simulink model "UpDownPendulum"  (Simulink 8.6)
settings: Solver=ode1  SolverMode=SingleTasking  StartTime=0.0  StopTime=200  FixedStep=0.001  RelTol=1e-3
undefined symbols (not defined in the file): Advantech, magnitude, PCI
libraries: sldrtlib x11, simulink x6
settings Model: Creator=Demo11  LastModifiedBy=demo  SimulationMode=external  ExtModeTrigMode=oneshot  ExtModeTrigDuration=100000
settings DataIOCC: LimitDataPoints=off  SignalLoggingName=sigsOut
settings OptimizationCC: BlockReduction=off  BooleanDataType=off  InitFltsAndDblsToZero=on
settings DebuggingCC: SaveWithParameterizedLinksMsg=none  SignalResolutionControl=TryResolveAllWithWarning  SolverPrmCheckMsg=none  MultiTaskDSMMsg=warning  MultiTaskCondExecSysMsg=none  FcnCallInpInsideContextMsg=UseLocalSettings
settings HardwareCC: ProdBitPerLong=64  ProdBitPerPointer=64  ProdIntDivRoundTo=Zero  ProdEndianess=LittleEndian  ProdWordSize=64  ProdHWDeviceType=Intel->x86-64  TargetBitPerLong=64  TargetBitPerPointer=64  TargetIntDivRoundTo=Zero  TargetEndianess=LittleEndian  TargetWordSize=64  TargetHWDeviceType=Intel->x86-64
settings RTWCC: SystemTargetFile=sldrt.tlc  TemplateMakefile=sldrt.tmf  Description=Simulink Desktop Real-Time  RTWCompilerOptimization=on
settings CodeAppCC: MaxIdLength=95
settings SimulinkDesktopRealTimeCC: TargetPreCompLibLocation=C:\Program Files\MATLAB\R2015b\toolbox\sldrt\lib\win64  TargetLangStandard=C89/C90 (ANSI)  SupportVariableSizeSignals=off

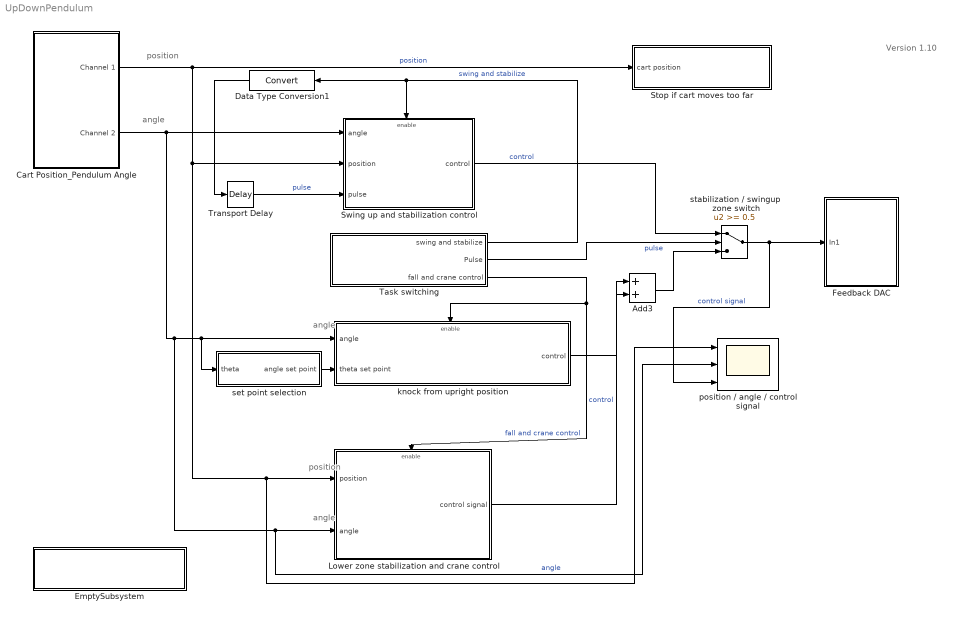
== system UpDownPendulum ==
  note: position
  note: angle
  note: Version 1.10
  note: angle
  note: angle
  note: position
  Add3 : Sum
  Cart Position_Pendulum Angle : Subsystem  mask(Feedback Encoder Block){st=0.001, of1=0, of2=-1024}
      mask prompts: st "Sample Time"; of1 "Channel 1 Offset"; of2 "Channel 2 Offset"
      mask help: Special block to use with the Feedback experiments to read encoder channels using the digital I/O lines
      mask Display:
      | image(imread('bckg.bmp'))
      | disp('PCI1711 \n Lab I/O Board \n\n\n Feedback Encoder')
  Data Type Conversion1 : DataTypeConversion
  EmptySubsystem : Subsystem
      mask Display:
      | image(imread('FB-inst-blue2.jpg'))
      | disp('\n\nFeedback Instruments Limited')
  Feedback DAC : Subsystem  mask(DAC Unit for Feedback Experiments){st=0.001, ch=1}
      mask prompts: st "Sample Time"; ch "Output Channel"
      mask help:
      | Digital to Analog Output  for Feedback Experiments
      | using Advantech PCI1711  I/O board
      mask Display:
      | image(imread('bckg.bmp'))
      | disp('PCI1711 \n Lab I/O Board \n\n Feedback  DAC \n for Pendulum')
  Lower zone stabilization and crane control : Subsystem  TreatAsAtomicUnit=on
      mask Display:
      | image(imread('bckg.bmp'))
      | disp('Lower zone stabilization \nand crane control')
  Stop if cart moves too far : Subsystem
      mask Display:
      | image(imread('bckg.bmp'))
      | disp('Stop if cart moves too far')
  Swing up and stabilization control : Subsystem  TreatAsAtomicUnit=on
      mask Display:
      | image(imread('bckg.bmp'))
      | disp('Swing up \nand stabilization control')
  Task switching : Subsystem
      mask Display:
      | image(imread('bckg.bmp'))
      | disp('Task switching')
  Transport Delay : TransportDelay  DelayTime=0.3  FixedBuffer=on
  knock from upright position : Subsystem  TreatAsAtomicUnit=on
      mask Display:
      | image(imread('bckg.bmp'))
      | disp('knock from upright position')
  position / angle / control signal : Scope  NumInputPorts=3
      mask Display: image(imread('scope.jpg'))
  set point selection : Subsystem
      mask Display:
      | image(imread('bckg.bmp'))
      | disp('Set point selection')
  stabilization / swingup  zone switch : Switch  Threshold=0.5
  wires:
  Cart Position_Pendulum Angle/1(Channel 1) -> Swing up and stabilization control/2(position), Lower zone stabilization and crane control/1(position), position / angle / control signal/1, Stop if cart moves too far/1(cart position)  "position"
  Cart Position_Pendulum Angle/2(Channel 2) -> knock from upright position/1(angle), set point selection/1(theta), Lower zone stabilization and crane control/2(angle), position / angle / control signal/2, Swing up and stabilization control/1(angle)  "angle"
  stabilization / swingup  zone switch/1 -> Feedback DAC/1(In1), position / angle / control signal/3  "control signal"
  Swing up and stabilization control/1(control) -> stabilization / swingup  zone switch/1  "control"
  set point selection/1(angle set point) -> knock from upright position/2(theta set point)
  Task switching/3(fall and crane control) -> knock from upright position/Enable, Lower zone stabilization and crane control/Enable  "fall and crane control"
  Add3/1 -> stabilization / swingup  zone switch/3
  Task switching/1(swing and stabilize) -> Swing up and stabilization control/Enable, Data Type Conversion1/1  "swing and stabilize"
  Transport Delay/1 -> Swing up and stabilization control/3(pulse)  "pulse"
  Data Type Conversion1/1 -> Transport Delay/1
  Task switching/2(Pulse) -> stabilization / swingup  zone switch/2  "pulse"
  Lower zone stabilization and crane control/1(control signal) -> Add3/2  "control"
  knock from upright position/1(control) -> Add3/1

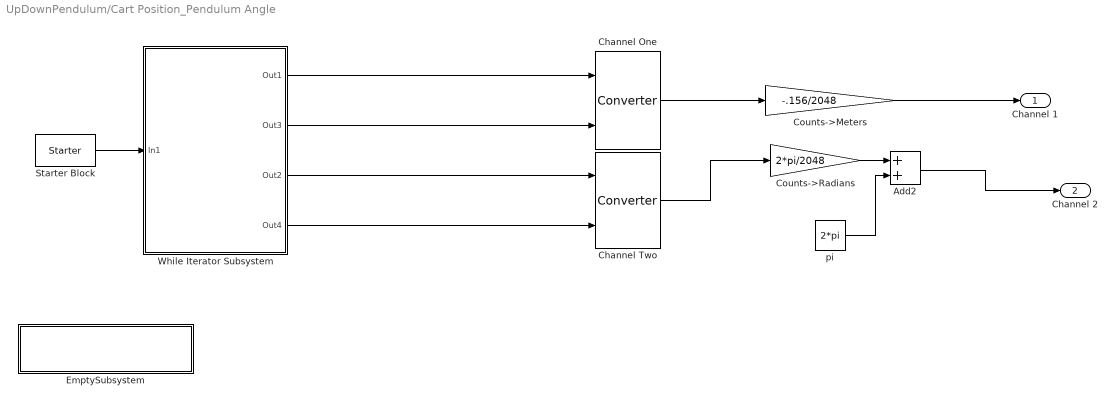
== system UpDownPendulum/Cart Position_Pendulum Angle ==
  Add2 : Sum
  Channel One : S-Function  FunctionName=Converter  Parameters=of1,st  SFunctionDeploymentMode=off  EnableBusSupport=off
  Channel Two : S-Function  FunctionName=Converter  Parameters=of2,st  SFunctionDeploymentMode=off  EnableBusSupport=off
  Counts->Meters : Gain  Gain=-.156/2048  SaturateOnIntegerOverflow=on  OutDataTypeStr=Inherit: Same as input  ParamDataTypeStr=Inherit: Same as input
  Counts->Radians : Gain  Gain=2*pi/2048  SaturateOnIntegerOverflow=on  OutDataTypeStr=Inherit: Same as input  ParamDataTypeStr=Inherit: Same as input
  EmptySubsystem : Subsystem
      mask Display:
      | image(imread('FB-inst-blue2.jpg'))
      | disp('\n\nFeedback Instruments Limited')
  Starter Block : S-Function  FunctionName=Starter  Parameters=sample_time  SFunctionDeploymentMode=off  EnableBusSupport=off  mask{sample_time=st}
      mask prompts: sample_time "Sample Time:"
  While Iterator Subsystem : Subsystem  TreatAsAtomicUnit=on
  pi : Constant  Value=2*pi
  Channel 1 : Outport
  Channel 2 : Outport  Port=2
  wires:
  Channel One/1 -> Counts->Meters/1
  While Iterator Subsystem/4(Out4) -> Channel Two/2
  While Iterator Subsystem/3(Out2) -> Channel Two/1
  While Iterator Subsystem/2(Out3) -> Channel One/2
  While Iterator Subsystem/1(Out1) -> Channel One/1
  Starter Block/1 -> While Iterator Subsystem/1(In1)
  Counts->Meters/1 -> Channel 1/1
  Counts->Radians/1 -> Add2/1
  pi/1 -> Add2/2
  Channel Two/1 -> Counts->Radians/1
  Add2/1 -> Channel 2/1

== system UpDownPendulum/EmptySubsystem ==

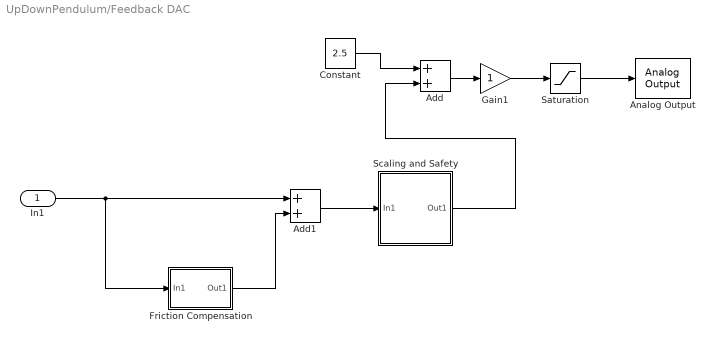
== system UpDownPendulum/Feedback DAC ==
  In1 : Inport
  Add : Sum  OutDataTypeStr=Inherit: Same as first input
  Add1 : Sum
  Analog Output : sldrtlib/Analog Output  SampleTime=st  MaxMissedTicks=10  ShowMissedTicks=off  YieldWhenWaiting=off  DrvName=Advantech/PCI-1711  DrvAddress=4294967295  DrvOptions=zeros(1,0)  Channels=ch  RangeMode=1  VoltRange=2  InitialValue=2.5  FinalValue=2.5
      settings: AttributesFormatString=Advantech\nPCI-1711 [auto]
  Constant : Constant  Value=2.5
  Friction Compensation : Subsystem  mask(linear){frictionCompNeg=.1, frictionCompPos=.1}
      mask prompts: frictionCompNeg "Friction Compensation Magnitude in Negative Direction"; frictionCompPos "Friction Compensation Magnitude in Positive Direction"
      mask Display: plot(0,0,100,100,[40,30,20],[87,85,80],[46,54,54,46,46],[90,90,80,80,90],[46,45,45,46,54,55,55,54,46],[78,80,90,91,91,90,80,78,78],[51,51,49,49],[78,10,10,78],[90,80,70,60],[70,80,85,88],[20,10],[80,70],[20,20,15],[73,80,80],[85,80,80],[80,80,74])
  Gain1 : Gain
  Saturation : Saturate  UpperLimit=5.0  LowerLimit=0
  Scaling and Safety : Subsystem
  wires:
  Add1/1 -> Scaling and Safety/1(In1)
  In1/1 -> Add1/1, Friction Compensation/1(In1)
  Friction Compensation/1(Out1) -> Add1/2
  Constant/1 -> Add/1
  Saturation/1 -> Analog Output/1
  Add/1 -> Gain1/1
  Gain1/1 -> Saturation/1
  Scaling and Safety/1(Out1) -> Add/2

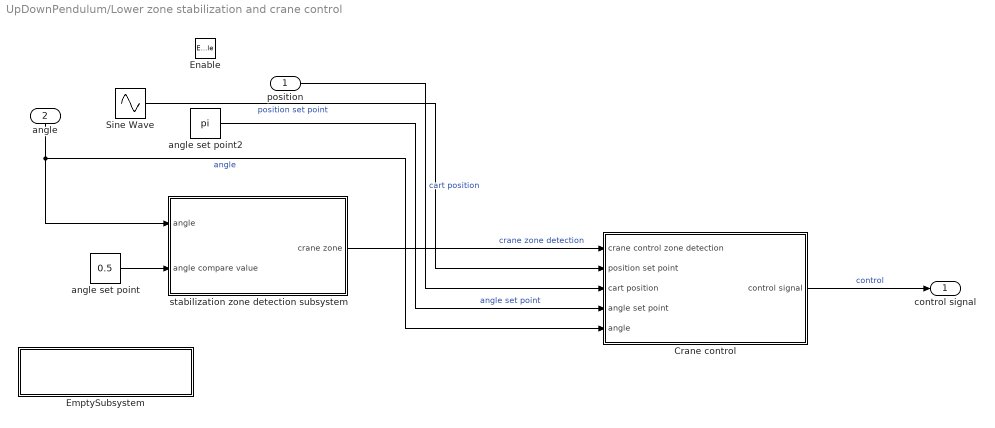
== system UpDownPendulum/Lower zone stabilization and crane control ==
  position : Inport
  angle : Inport  Port=2
  Enable : EnablePort
  Crane control : Subsystem
      mask Display:
      | image(imread('bckg.bmp'))
      | disp('Crane control')
  EmptySubsystem : Subsystem
      mask Display:
      | image(imread('FB-inst-blue2.jpg'))
      | disp('\n\nFeedback Instruments Limited')
  Sine Wave : Sin  Amplitude=0.1  Frequency=2  SampleTime=0
  angle set point : Constant  Value=0.5
  angle set point2 : Constant  Value=pi
  stabilization zone detection subsystem : Subsystem
      mask Display:
      | image(imread('bckg.bmp'))
      | disp('Stabilization zone \ndetection system')
  control signal : Outport
  wires:
  angle set point2/1 -> Crane control/4(angle set point)  "angle set point"
  angle set point/1 -> stabilization zone detection subsystem/2(angle compare value)
  stabilization zone detection subsystem/1(crane zone) -> Crane control/1(crane control zone detection)  "crane zone detection"
  angle/1 -> stabilization zone detection subsystem/1(angle), Crane control/5(angle)  "angle"
  Crane control/1(control signal) -> control signal/1  "control"
  Sine Wave/1 -> Crane control/2(position set point)  "position set point"
  position/1 -> Crane control/3(cart position)  "cart position"

== system UpDownPendulum/Stop if cart moves too far ==
  cart position : Inport
  Abs3 : Abs
  Compare To Constant1 : simulink/Logic and Bit Operations/Compare To Constant  relop=>  const=0.4  OutDataTypeStr=boolean  ZeroCross=off
  Data Type Conversion1 : DataTypeConversion
  Stop Simulation if cart moves to far : Stop
  wires:
  cart position/1 -> Abs3/1
  Data Type Conversion1/1 -> Stop Simulation if cart moves to far/1
  Compare To Constant1/1 -> Data Type Conversion1/1
  Abs3/1 -> Compare To Constant1/1

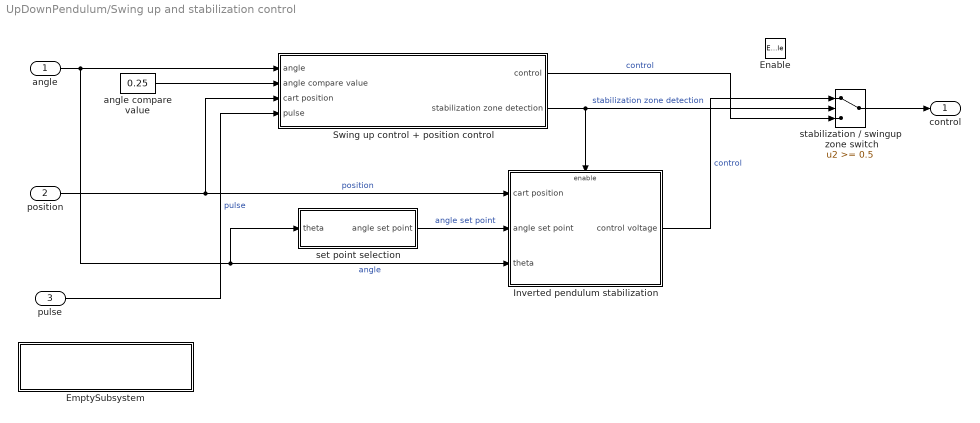
== system UpDownPendulum/Swing up and stabilization control ==
  angle : Inport
  position : Inport  Port=2
  pulse : Inport  Port=3
  Enable : EnablePort
  EmptySubsystem : Subsystem
      mask Display:
      | image(imread('FB-inst-blue2.jpg'))
      | disp('\n\nFeedback Instruments Limited')
  Inverted pendulum stabilization : Subsystem  TreatAsAtomicUnit=on
      mask Display:
      | image(imread('bckg.bmp'))
      | disp('Inverted pendulum \nstabilization')
  Swing up control + position control : Subsystem
      mask Display:
      | image(imread('bckg.bmp'))
      | disp('Swing up control \nand position control')
  angle compare value : Constant  Value=0.25
  set point selection : Subsystem
      mask Display:
      | image(imread('bckg.bmp'))
      | disp('Set point selection')
  stabilization / swingup  zone switch : Switch  Threshold=0.5
  control : Outport
  wires:
  angle/1 -> Swing up control + position control/1(angle), set point selection/1(theta), Inverted pendulum stabilization/3(theta)  "angle"
  Swing up control + position control/1(control) -> stabilization / swingup  zone switch/3  "control"
  Inverted pendulum stabilization/1(control voltage) -> stabilization / swingup  zone switch/1  "control"
  set point selection/1(angle set point) -> Inverted pendulum stabilization/2(angle set point)  "angle set point"
  Swing up control + position control/2(stabilization zone detection) -> stabilization / swingup  zone switch/2, Inverted pendulum stabilization/Enable  "stabilization zone detection"
  angle compare value/1 -> Swing up control + position control/2(angle compare value)
  position/1 -> Inverted pendulum stabilization/1(cart position), Swing up control + position control/3(cart position)  "position"
  stabilization / swingup  zone switch/1 -> control/1
  pulse/1 -> Swing up control + position control/4(pulse)  "pulse"

== system UpDownPendulum/Task switching ==
  Compare To Constant : simulink/Logic and Bit Operations/Compare To Constant  relop=<  const=0.5  OutDataTypeStr=boolean  ZeroCross=off
  Compare To Constant1 : simulink/Logic and Bit Operations/Compare To Constant  relop=>  const=0.5  OutDataTypeStr=boolean  ZeroCross=off
  Pulse Generator : DiscretePulseGenerator  PulseType=Time based  Period=60  PulseWidth=50
  swing and stabilize : Outport
  Pulse : Outport  Port=2
  fall and crane control : Outport  Port=3
  wires:
  Pulse Generator/1 -> Compare To Constant/1, Compare To Constant1/1, Pulse/1
  Compare To Constant1/1 -> swing and stabilize/1
  Compare To Constant/1 -> fall and crane control/1

== system UpDownPendulum/knock from upright position ==
  angle : Inport
  theta set point : Inport  Port=2
  Enable : EnablePort
  control v : Constant  Value=0
  first pendulum move : Switch  Threshold=0.2
  kick pendulum out of stand on proper side : Subsystem
  control : Outport
  wires:
  angle/1 -> kick pendulum out of stand on proper side/1(angle)
  control v/1 -> first pendulum move/1
  first pendulum move/1 -> control/1
  theta set point/1 -> kick pendulum out of stand on proper side/2(angle set point)
  kick pendulum out of stand on proper side/1(angle deviation form horizontal position) -> first pendulum move/2
  kick pendulum out of stand on proper side/2(contol voltage pulse) -> first pendulum move/3

== system UpDownPendulum/set point selection ==
  theta : Inport
  0 : Constant  Value=0
  2*pi : Constant  Value=2*pi
  Abs : Abs
  zero velocity : Switch  Threshold=pi
  angle set point : Outport
  wires:
  zero velocity/1 -> angle set point/1
  theta/1 -> Abs/1
  Abs/1 -> zero velocity/2
  2*pi/1 -> zero velocity/1
  0/1 -> zero velocity/3

== system UpDownPendulum/Cart Position_Pendulum Angle/EmptySubsystem ==

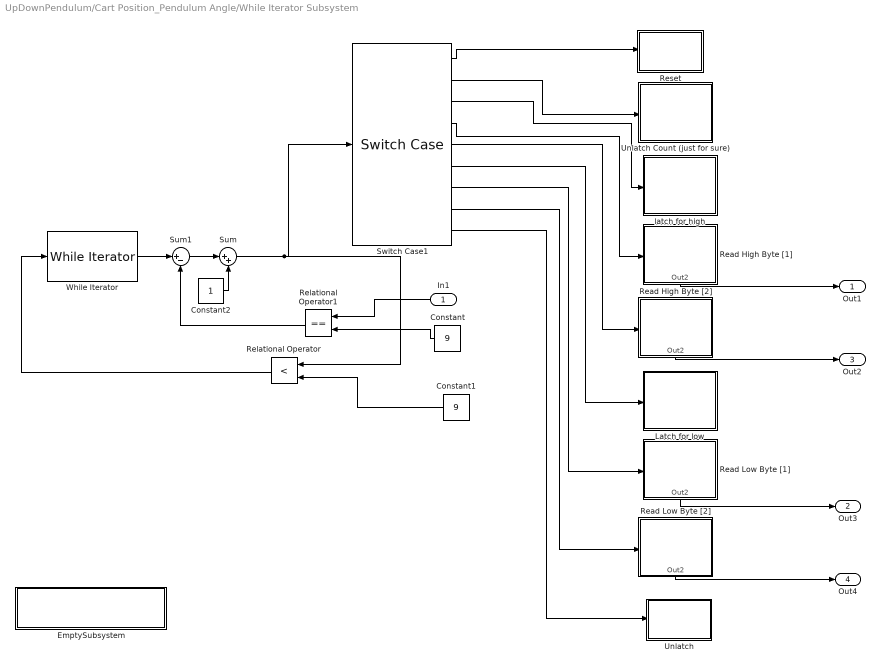
== system UpDownPendulum/Cart Position_Pendulum Angle/While Iterator Subsystem ==
  In1 : Inport
  Constant : Constant  Value=9
  Constant1 : Constant  Value=9
  Constant2 : Constant
  EmptySubsystem : Subsystem
      mask Display:
      | image(imread('FB-inst-blue2.jpg'))
      | disp('\n\nFeedback Instruments Limited')
  Latch for low : Subsystem  TreatAsAtomicUnit=on
  Read High Byte [1] : Subsystem  TreatAsAtomicUnit=on
  Read High Byte [2] : Subsystem  TreatAsAtomicUnit=on
  Read Low Byte [1] : Subsystem  TreatAsAtomicUnit=on
  Read Low Byte [2] : Subsystem  TreatAsAtomicUnit=on
  Relational Operator : RelationalOperator  Operator=<  OutDataTypeStr=boolean
  Relational Operator1 : RelationalOperator  Operator===  OutDataTypeStr=boolean
  Reset : Subsystem  TreatAsAtomicUnit=on
  Sum : Sum  Inputs=|++
  Sum1 : Sum  Inputs=|+-  OutDataTypeStr=Inherit: Same as first input
  Switch Case1 : SwitchCase  CaseConditions={1,2,3,4,5,6,7,8,9}  ShowDefaultCase=off
  Unlatch : Subsystem  TreatAsAtomicUnit=on
  "Unlatch Count (just for sure) " : Subsystem  TreatAsAtomicUnit=on
  While Iterator : WhileIterator  MaxIters=9  WhileBlockType=do-while  ResetStates=reset  ShowIterationPort=on  OutputDataType=int8
  latch for high : Subsystem  TreatAsAtomicUnit=on
  Out1 : Outport
  Out3 : Outport  Port=2
  Out2 : Outport  Port=3
  Out4 : Outport  Port=4
  wires:
  Switch Case1/9 -> Unlatch/Action
  Switch Case1/8 -> Read Low Byte [2]/Action
  Switch Case1/7 -> Read Low Byte [1]/Action
  Switch Case1/6 -> Latch for low/Action
  Switch Case1/5 -> Read High Byte [2]/Action
  Switch Case1/4 -> Read High Byte [1]/Action
  Switch Case1/3 -> latch for high/Action
  Constant2/1 -> Sum/2
  Sum/1 -> Relational Operator/1, Switch Case1/1
  Sum1/1 -> Sum/1
  Read Low Byte [2]/1(Out2) -> Out4/1
  Read Low Byte [1]/1(Out2) -> Out3/1
  Read High Byte [2]/1(Out2) -> Out2/1
  Read High Byte [1]/1(Out2) -> Out1/1
  Constant1/1 -> Relational Operator/2
  Switch Case1/2 -> "Unlatch Count (just for sure) "/Action
  Switch Case1/1 -> Reset/Action
  While Iterator/1 -> Sum1/1
  Relational Operator1/1 -> Sum1/2
  Constant/1 -> Relational Operator1/2
  In1/1 -> Relational Operator1/1
  Relational Operator/1 -> While Iterator/1

== system UpDownPendulum/Feedback DAC/Friction Compensation ==
  In1 : Inport
  " " : Gain  Gain=frictionCompPos  SaturateOnIntegerOverflow=on  OutDataTypeStr=Inherit: Same as input  ParamDataTypeStr=Inherit: Same as input
  3 : Switch  SaturateOnIntegerOverflow=on  InputSameDT=on
  Gain3 : Gain  Gain=frictionCompNeg  SaturateOnIntegerOverflow=on  OutDataTypeStr=Inherit: Same as input  ParamDataTypeStr=Inherit: Same as input
  Sign2 : Signum  Tag=T
  Out1 : Outport  InitialOutput=0
  wires:
  3/1 -> Out1/1
  Sign2/1 -> 3/2, " "/1, Gain3/1
  Gain3/1 -> 3/3
  " "/1 -> 3/1
  In1/1 -> Sign2/1

== system UpDownPendulum/Feedback DAC/Scaling and Safety ==
  In1 : Inport
  -1 : Gain  Gain=-1  SaturateOnIntegerOverflow=on  OutDataTypeStr=Inherit: Same as input  ParamDataTypeStr=Inherit: Same as input
  Saturation : Saturate  UpperLimit=2.5  LowerLimit=-2.5
  Out1 : Outport
  wires:
  -1/1 -> Saturation/1  "actual LoadPosition"
  In1/1 -> -1/1
  Saturation/1 -> Out1/1

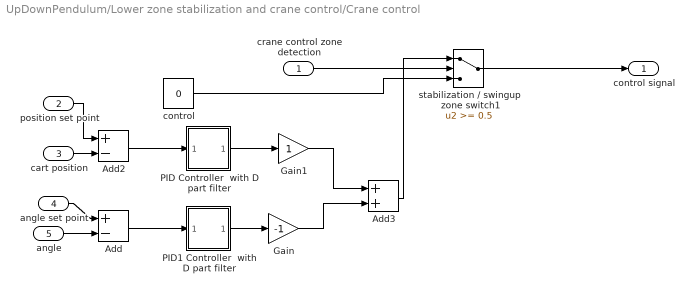
== system UpDownPendulum/Lower zone stabilization and crane control/Crane control ==
  crane control zone detection : Inport
  position set point : Inport  Port=2
  cart position : Inport  Port=3
  angle set point : Inport  Port=4
  angle : Inport  Port=5
  Add : Sum  Inputs=+-
  Add2 : Sum  Inputs=+-
  Add3 : Sum
  Gain : Gain  Gain=-1
  Gain1 : Gain
  PID Controller  with D part filter : Subsystem  AncestorBlock=simulink_extras/Additional Linear/PID Controller  mask(PID Controller){P=7, I=2, D=1}
      mask prompts: P "Proportional:"; I "Integral:"; D "Derivative:"
      mask help:
      | Enter expressions for proportional, integral, and derivative terms.
      | P+I/s+Ds
      mask Help: This block implements a PID controller where parameters are entered for the Proportional, Integral and Derivative terms. Unmask this block to see how it works. The derivative term is implemented using a true derivative block.
      mask Callback P:
      | if str2num(get_param(gcb, 'P'))>10
      |  WARNDLG('Proportional Gain is out of the range [3..10] and is set to maximum value now', 'Setting Value Error')
      |  set_param(gcb,'P','10');
      | end
      | if str2num(get_param(gcb, 'P'))<3
      |  WARNDLG('Proportional Gain is out of the range [3..10] and is set to minimum now', 'Setting Value Error')
      |  set_param(gcb,'P','3');
      | end
      mask Callback I:
      | if str2num(get_param(gcb, 'I'))>3
      |  WARNDLG('Integral Gain is out of the range [1..3] and is set to maximum value now', 'Setting Value Error')
      |  set_param(gcb,'I','3');
      | end
      | if str2num(get_param(gcb, 'I'))<1
      |  WARNDLG('Integral Gain is out of the range [1..3] and is set to minimum now', 'Setting Value Error')
      |  set_param(gcb,'I','1');
      | end
      mask Callback D:
      | if str2num(get_param(gcb, 'D'))>3
      |  WARNDLG('Derivative Gain is out of the range [1..3] and is set to maximum value now', 'Setting Value Error')
      |  set_param(gcb,'D','3');
      | end
      | if str2num(get_param(gcb, 'D'))<1
      |  WARNDLG('Derivative Gain is out of the range [1..3] and is set to minimum now', 'Setting Value Error')
      |  set_param(gcb,'D','1');
      | end
      mask Display:
      | image(imread('bckg.bmp'))
      | disp('PID')
  PID1 Controller  with D part filter : Subsystem  AncestorBlock=simulink_extras/Additional Linear/PID Controller  mask(PID Controller){P=4, I=0, D=0.1}
      mask prompts: P "Proportional:"; I "Integral:"; D "Derivative:"
      mask help:
      | Enter expressions for proportional, integral, and derivative terms.
      | P+I/s+Ds
      mask Help: This block implements a PID controller where parameters are entered for the Proportional, Integral and Derivative terms. Unmask this block to see how it works. The derivative term is implemented using a true derivative block.
      mask Callback P:
      | if str2num(get_param(gcb, 'P'))>6
      |  WARNDLG('Proportional Gain is out of the range [2..6] and is set to maximum value now', 'Setting Value Error')
      |  set_param(gcb,'P','6');
      | end
      | if str2num(get_param(gcb, 'P'))<2
      |  WARNDLG('Proportional Gain is out of the range [2..6] and is set to minimum now', 'Setting Value Error')
      |  set_param(gcb,'P','2');
      | end
      mask Callback I:
      | if str2num(get_param(gcb, 'I'))>0.1
      |  WARNDLG('Integral Gain is out of the range [-0.1 .. 0.1] and is set to maximum value now', 'Setting Value Error')
      |  set_param(gcb,'I','0.1');
      | end
      | if str2num(get_param(gcb, 'I'))<-0.1
      |  WARNDLG('Integral Gain is out of the range [-0.1 .. 0.1] and is set to minimum now', 'Setting Value Error')
      |  set_param(gcb,'I','-0.1');
      | end
      mask Callback D:
      | if str2num(get_param(gcb, 'D'))>0.15
      |  WARNDLG('Derivative Gain is out of the range [0.05 .. 0.15] and is set to maximum value now', 'Setting Value Error')
      |  set_param(gcb,'D','0.15');
      | end
      | if str2num(get_param(gcb, 'D'))<0.05
      |  WARNDLG('Derivative Gain is out of the range [0.05 .. 0.15] and is set to minimum now', 'Setting Value Error')
      |  set_param(gcb,'D','0.05');
      | end
      mask Display:
      | image(imread('bckg.bmp'))
      | disp('PID')
  control : Constant  Value=0
  stabilization / swingup  zone switch1 : Switch  Threshold=0.5
  control signal : Outport
  wires:
  PID1 Controller  with D part filter/1(Out_1) -> Gain/1
  Gain/1 -> Add3/2
  Add/1 -> PID1 Controller  with D part filter/1(In_1)
  Add2/1 -> PID Controller  with D part filter/1(In_1)
  PID Controller  with D part filter/1(Out_1) -> Gain1/1
  control/1 -> stabilization / swingup  zone switch1/3
  Gain1/1 -> Add3/1
  Add3/1 -> stabilization / swingup  zone switch1/1
  angle/1 -> Add/2
  crane control zone detection/1 -> stabilization / swingup  zone switch1/2
  stabilization / swingup  zone switch1/1 -> control signal/1
  position set point/1 -> Add2/1
  cart position/1 -> Add2/2
  angle set point/1 -> Add/1

== system UpDownPendulum/Lower zone stabilization and crane control/EmptySubsystem ==

== system UpDownPendulum/Lower zone stabilization and crane control/stabilization zone detection subsystem ==
  angle : Inport
  angle compare value : Inport  Port=2
  Add1 : Sum  Inputs=+-
  Add2 : Sum
  Constant : Constant  Value=pi
  Logical Operator : Logic  AllPortsSameDT=off  OutDataTypeStr=boolean
  Relational Operator : RelationalOperator  Operator=>  OutDataTypeStr=boolean
  Relational Operator1 : RelationalOperator  Operator=<  OutDataTypeStr=boolean
  crane zone : Outport
  wires:
  Relational Operator1/1 -> Logical Operator/2
  Relational Operator/1 -> Logical Operator/1
  angle/1 -> Relational Operator1/1, Relational Operator/1
  Logical Operator/1 -> crane zone/1
  angle compare value/1 -> Add2/2, Add1/2
  Add2/1 -> Relational Operator1/2
  Constant/1 -> Add2/1, Add1/1
  Add1/1 -> Relational Operator/2

== system UpDownPendulum/Swing up and stabilization control/EmptySubsystem ==

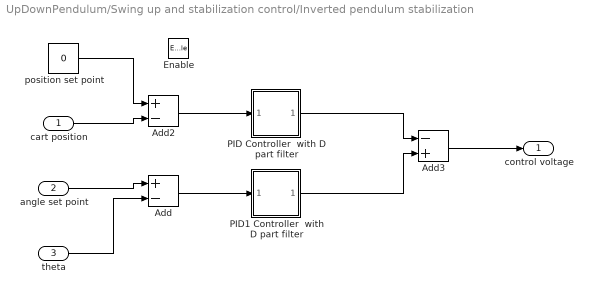
== system UpDownPendulum/Swing up and stabilization control/Inverted pendulum stabilization ==
  cart position : Inport
  angle set point : Inport  Port=2
  theta : Inport  Port=3
  Enable : EnablePort
  Add : Sum  Inputs=+-
  Add2 : Sum  Inputs=+-
  Add3 : Sum  Inputs=-+
  PID Controller  with D part filter : Subsystem  AncestorBlock=simulink_extras/Additional Linear/PID Controller  mask(PID Controller){P=7, I=0.5, D=3}
      mask prompts: P "Proportional:"; I "Integral:"; D "Derivative:"
      mask help:
      | Enter expressions for proportional, integral, and derivative terms.
      | P+I/s+Ds
      mask Help: This block implements a PID controller where parameters are entered for the Proportional, Integral and Derivative terms. Unmask this block to see how it works. The derivative term is implemented using a true derivative block.
      mask Callback P:
      | if str2num(get_param(gcb, 'P'))>10
      |  WARNDLG('Proportional Gain is out of the range [4..10] and is set to maximum value now', 'Setting Value Error')
      |  set_param(gcb,'P','10');
      | end
      | if str2num(get_param(gcb, 'P'))<4
      |  WARNDLG('Proportional Gain is out of the range [4..10] and is set to minimum now', 'Setting Value Error')
      |  set_param(gcb,'P','4');
      | end
      mask Callback I:
      | if str2num(get_param(gcb, 'I'))>0.75
      |  WARNDLG('Integral Gain is out of the range [0.25 .. 0.75] and is set to maximum value now', 'Setting Value Error')
      |  set_param(gcb,'I','0.75');
      | end
      | if str2num(get_param(gcb, 'I'))<0.25
      |  WARNDLG('Integral Gain is out of the range [0.25 .. 0.75] and is set to minimum now', 'Setting Value Error')
      |  set_param(gcb,'I','0.25');
      | end
      mask Callback D:
      | if str2num(get_param(gcb, 'D'))>5
      |  WARNDLG('Derivative Gain is out of the range [1..5] and is set to maximum value now', 'Setting Value Error')
      |  set_param(gcb,'D','5');
      | end
      | if str2num(get_param(gcb, 'D'))<1
      |  WARNDLG('Derivative Gain is out of the range [1..5] and is set to minimum now', 'Setting Value Error')
      |  set_param(gcb,'D','1');
      | end
      mask Display:
      | image(imread('bckg.bmp'))
      | disp('PID')
  PID1 Controller  with D part filter : Subsystem  AncestorBlock=simulink_extras/Additional Linear/PID Controller  mask(PID Controller){P=25, I=0.2, D=2}
      mask prompts: P "Proportional:"; I "Integral:"; D "Derivative:"
      mask help:
      | Enter expressions for proportional, integral, and derivative terms.
      | P+I/s+Ds
      mask Help: This block implements a PID controller where parameters are entered for the Proportional, Integral and Derivative terms. Unmask this block to see how it works. The derivative term is implemented using a true derivative block.
      mask Callback P:
      | if str2num(get_param(gcb, 'P'))>40
      |  WARNDLG('Proportional Gain is out of the range [10..40] and is set to maximum value now', 'Setting Value Error')
      |  set_param(gcb,'P','40');
      | end
      | if str2num(get_param(gcb, 'P'))<10
      |  WARNDLG('Proportional Gain is out of the range [10..40] and is set to minimum now', 'Setting Value Error')
      |  set_param(gcb,'P','10');
      | end
      mask Callback I:
      | if str2num(get_param(gcb, 'I'))>0.3
      |  WARNDLG('Integral Gain is out of the range [0.1 .. 0.3] and is set to maximum value now', 'Setting Value Error')
      |  set_param(gcb,'I','0.3');
      | end
      | if str2num(get_param(gcb, 'I'))<0.1
      |  WARNDLG('Integral Gain is out of the range [0.1 .. 0.3] and is set to minimum now', 'Setting Value Error')
      |  set_param(gcb,'I','0.1');
      | end
      mask Callback D:
      | if str2num(get_param(gcb, 'D'))>3
      |  WARNDLG('Derivative Gain is out of the range [1..3] and is set to maximum value now', 'Setting Value Error')
      |  set_param(gcb,'D','3');
      | end
      | if str2num(get_param(gcb, 'D'))<1
      |  WARNDLG('Derivative Gain is out of the range [1..3] and is set to minimum now', 'Setting Value Error')
      |  set_param(gcb,'D','1');
      | end
      mask Display:
      | image(imread('bckg.bmp'))
      | disp('PID')
  position set point : Constant  Value=0
  control voltage : Outport
  wires:
  PID1 Controller  with D part filter/1(Out_1) -> Add3/2
  Add/1 -> PID1 Controller  with D part filter/1(In_1)
  position set point/1 -> Add2/1
  Add2/1 -> PID Controller  with D part filter/1(In_1)
  PID Controller  with D part filter/1(Out_1) -> Add3/1
  cart position/1 -> Add2/2
  theta/1 -> Add/2
  angle set point/1 -> Add/1
  Add3/1 -> control voltage/1

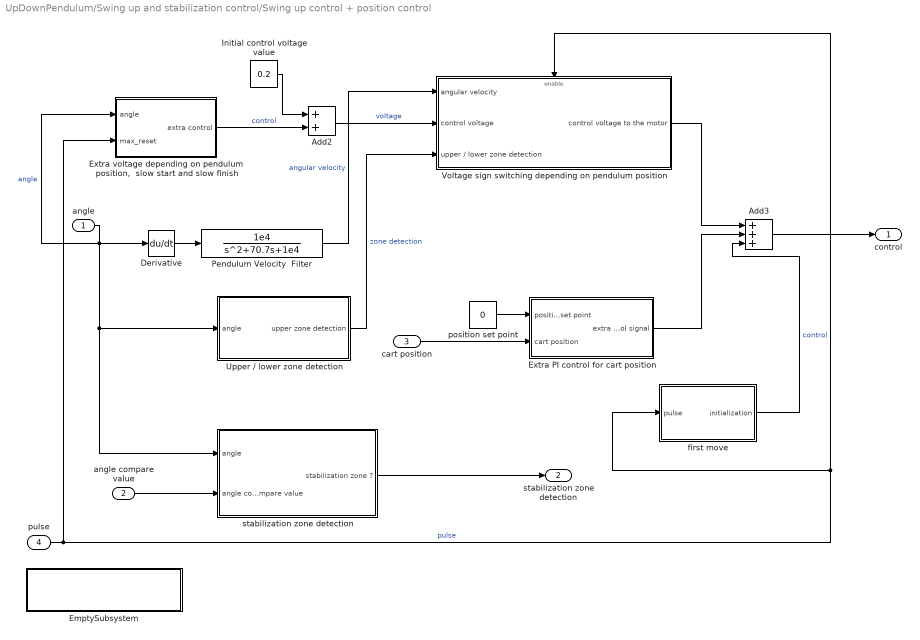
== system UpDownPendulum/Swing up and stabilization control/Swing up control + position control ==
  angle : Inport
  angle compare value : Inport  Port=2
  cart position : Inport  Port=3
  pulse : Inport  Port=4
  Add2 : Sum
  Add3 : Sum  Inputs=+++
  Derivative : Derivative
  EmptySubsystem : Subsystem
      mask Display:
      | image(imread('FB-inst-blue2.jpg'))
      | disp('\n\nFeedback Instruments Limited')
  Extra PI control for cart position : Subsystem
  "Extra voltage depending on pendulum position,  slow start and slow finish" : Subsystem
      mask Display:
      | image(imread('bckg.bmp'))
      | disp('Extra voltage')
  Initial control voltage value : Constant  Value=0.2
  Pendulum Velocity  Filter : TransferFcn  Numerator=[1e4]  Denominator=[1 70.7 1e4]
  Upper / lower zone detection : Subsystem
      mask Display:
      | image(imread('bckg.bmp'))
      | disp('Upper / lower zone \ndetection')
  Voltage sign switching depending on pendulum position : Subsystem  TreatAsAtomicUnit=on
      mask Display:
      | image(imread('bckg.bmp'))
      | disp('Voltage sign switching \ndepending on pendulum position')
  first move : Subsystem
      mask Display:
      | image(imread('bckg.bmp'))
      | disp('First move')
  position set point : Constant  Value=0
  "stabilization zone detection " : Subsystem
      mask Display:
      | image(imread('bckg.bmp'))
      | disp('stabilization zone detection')
  control : Outport
  stabilization zone detection : Outport  Port=2
  wires:
  Upper / lower zone detection/1(upper zone detection) -> Voltage sign switching depending on pendulum position/3(upper / lower zone detection)  "zone detection"
  Initial control voltage value/1 -> Add2/1
  Add2/1 -> Voltage sign switching depending on pendulum position/2(control voltage)  "voltage"
  angle/1 -> "Extra voltage depending on pendulum position,  slow start and slow finish"/1(angle), Derivative/1, "stabilization zone detection "/1(angle), Upper / lower zone detection/1(angle)  "angle"
  Derivative/1 -> Pendulum Velocity  Filter/1
  Pendulum Velocity  Filter/1 -> Voltage sign switching depending on pendulum position/1(angular velocity)  "angular velocity"
  "stabilization zone detection "/1(stabilization zone ?) -> stabilization zone detection/1
  angle compare value/1 -> "stabilization zone detection "/2(angle compare value)
  position set point/1 -> Extra PI control for cart position/1(position set point)
  cart position/1 -> Extra PI control for cart position/2(cart position)
  Extra PI control for cart position/1(extra control signal) -> Add3/2
  Voltage sign switching depending on pendulum position/1(control voltage to the motor) -> Add3/1
  Add3/1 -> control/1
  pulse/1 -> Voltage sign switching depending on pendulum position/Enable, first move/1(pulse), "Extra voltage depending on pendulum position,  slow start and slow finish"/2(max_reset)  "pulse"
  first move/1(initialization) -> Add3/3  "control"
  "Extra voltage depending on pendulum position,  slow start and slow finish"/1(extra control) -> Add2/2  "control"

== system UpDownPendulum/Swing up and stabilization control/set point selection ==
  theta : Inport
  0 : Constant  Value=0
  2*pi : Constant  Value=2*pi
  Abs : Abs
  zero velocity : Switch  Threshold=pi
  angle set point : Outport
  wires:
  zero velocity/1 -> angle set point/1
  theta/1 -> Abs/1
  Abs/1 -> zero velocity/2
  2*pi/1 -> zero velocity/1
  0/1 -> zero velocity/3

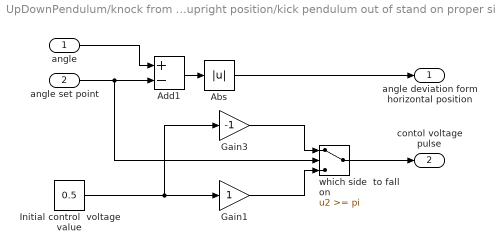
== system UpDownPendulum/knock from upright position/kick pendulum out of stand on proper side ==
  angle : Inport
  angle set point : Inport  Port=2
  Abs : Abs
  Add1 : Sum  Inputs=+-
  Gain1 : Gain
  Gain3 : Gain  Gain=-1
  Initial control  voltage value : Constant  Value=0.5
  which side  to fall on : Switch  Threshold=pi
  angle deviation form horizontal position : Outport
  contol voltage pulse : Outport  Port=2
  wires:
  angle set point/1 -> Add1/2, which side  to fall on/2
  Initial control  voltage value/1 -> Gain3/1, Gain1/1
  Gain3/1 -> which side  to fall on/1
  Gain1/1 -> which side  to fall on/3
  Add1/1 -> Abs/1
  angle/1 -> Add1/1
  which side  to fall on/1 -> contol voltage pulse/1
  Abs/1 -> angle deviation form horizontal position/1

== system UpDownPendulum/Cart Position_Pendulum Angle/While Iterator Subsystem/EmptySubsystem ==

== system UpDownPendulum/Cart Position_Pendulum Angle/While Iterator Subsystem/Latch for low ==
  Action Port : ActionPort  ActionType=case
  Constant : Constant  Value=6  OutDataTypeStr=double
  Digital Output : sldrtlib/Digital Output  SampleTime=-1  MaxMissedTicks=10  ShowMissedTicks=off  YieldWhenWaiting=off  DrvName=Advantech/PCI-1711  DrvAddress=4294967295  DrvOptions=zeros(1,0)  Channels=1  BitMode=2  InitialValue=0  FinalValue=0
      settings: AttributesFormatString=Advantech\nPCI-1711 [auto]
  wires:
  Constant/1 -> Digital Output/1

== system UpDownPendulum/Cart Position_Pendulum Angle/While Iterator Subsystem/Read High Byte [1] ==
  Action Port : ActionPort  ActionType=case
  Constant1 : Constant  Value=[1 2 4 8 16 32 64 128]
  Digital Input1 : sldrtlib/Digital Input  SampleTime=-1  MaxMissedTicks=10  ShowMissedTicks=off  YieldWhenWaiting=off  DrvName=Advantech/PCI-1711  DrvAddress=4294967295  DrvOptions=zeros(1,0)  Channels=[1,2,3,4,5,6,7,8]  BitMode=1  DataType=1
      settings: AttributesFormatString=Advantech\nPCI-1711 [auto]
  Dot Product : DotProduct  InputSameDT=on  OutDataTypeStr=Inherit: Inherit via internal rule
  Out2 : Outport
  wires:
  Digital Input1/1 -> Dot Product/1
  Constant1/1 -> Dot Product/2
  Dot Product/1 -> Out2/1

== system UpDownPendulum/Cart Position_Pendulum Angle/While Iterator Subsystem/Read High Byte [2] ==
  Action Port : ActionPort  ActionType=case
  Constant1 : Constant  Value=[1 2 4 8 16 32 64 128]
  Digital Input1 : sldrtlib/Digital Input  SampleTime=-1  MaxMissedTicks=10  ShowMissedTicks=off  YieldWhenWaiting=off  DrvName=Advantech/PCI-1711  DrvAddress=4294967295  DrvOptions=zeros(1,0)  Channels=[9:16]  BitMode=1  DataType=1
      settings: AttributesFormatString=Advantech\nPCI-1711 [auto]
  Dot Product : DotProduct  InputSameDT=on  OutDataTypeStr=Inherit: Inherit via internal rule
  Out2 : Outport
  wires:
  Dot Product/1 -> Out2/1
  Constant1/1 -> Dot Product/2
  Digital Input1/1 -> Dot Product/1

== system UpDownPendulum/Cart Position_Pendulum Angle/While Iterator Subsystem/Read Low Byte [1] ==
  Action Port : ActionPort  ActionType=case
  Constant1 : Constant  Value=[1 2 4 8 16 32 64 128]
  Digital Input1 : sldrtlib/Digital Input  SampleTime=-1  MaxMissedTicks=10  ShowMissedTicks=off  YieldWhenWaiting=off  DrvName=Advantech/PCI-1711  DrvAddress=4294967295  DrvOptions=zeros(1,0)  Channels=[1:8]  BitMode=1  DataType=1
      settings: AttributesFormatString=Advantech\nPCI-1711 [auto]
  Dot Product : DotProduct  InputSameDT=on  OutDataTypeStr=Inherit: Inherit via internal rule
  Out2 : Outport
  wires:
  Dot Product/1 -> Out2/1
  Constant1/1 -> Dot Product/2
  Digital Input1/1 -> Dot Product/1

== system UpDownPendulum/Cart Position_Pendulum Angle/While Iterator Subsystem/Read Low Byte [2] ==
  Action Port : ActionPort  ActionType=case
  Constant1 : Constant  Value=[1 2 4 8 16 32 64 128]
  Digital Input1 : sldrtlib/Digital Input  SampleTime=-1  MaxMissedTicks=10  ShowMissedTicks=off  YieldWhenWaiting=off  DrvName=Advantech/PCI-1711  DrvAddress=4294967295  DrvOptions=zeros(1,0)  Channels=[9:16]  BitMode=1  DataType=1
      settings: AttributesFormatString=Advantech\nPCI-1711 [auto]
  Dot Product : DotProduct  InputSameDT=on  OutDataTypeStr=Inherit: Inherit via internal rule
  Out2 : Outport
  wires:
  Dot Product/1 -> Out2/1
  Digital Input1/1 -> Dot Product/1
  Constant1/1 -> Dot Product/2

== system UpDownPendulum/Cart Position_Pendulum Angle/While Iterator Subsystem/Reset ==
  Action Port : ActionPort  ActionType=case
  Constant : Constant  Value=3  OutDataTypeStr=double
  Digital Output1 : sldrtlib/Digital Output  SampleTime=-1  MaxMissedTicks=10  ShowMissedTicks=off  YieldWhenWaiting=off  DrvName=Advantech/PCI-1711  DrvAddress=4294967295  DrvOptions=zeros(1,0)  Channels=1  BitMode=2  InitialValue=0  FinalValue=0
      settings: AttributesFormatString=Advantech\nPCI-1711 [auto]
  Subsystem : Subsystem
  wires:
  Subsystem/1(Out1) -> Digital Output1/1
  Constant/1 -> Subsystem/1(In1)

== system UpDownPendulum/Cart Position_Pendulum Angle/While Iterator Subsystem/Unlatch ==
  Action Port : ActionPort  ActionType=case
  Constant : Constant  Value=7  OutDataTypeStr=double
  Digital Output1 : sldrtlib/Digital Output  SampleTime=-1  MaxMissedTicks=10  ShowMissedTicks=off  YieldWhenWaiting=off  DrvName=Advantech/PCI-1711  DrvAddress=4294967295  DrvOptions=zeros(1,0)  Channels=1  BitMode=2  InitialValue=0  FinalValue=0
      settings: AttributesFormatString=Advantech\nPCI-1711 [auto]
  wires:
  Constant/1 -> Digital Output1/1

== system UpDownPendulum/Cart Position_Pendulum Angle/While Iterator Subsystem/Unlatch Count (just for sure)  ==
  Action Port : ActionPort  ActionType=case
  Constant : Constant  Value=7  OutDataTypeStr=double
  Digital Output : sldrtlib/Digital Output  SampleTime=-1  MaxMissedTicks=10  ShowMissedTicks=off  YieldWhenWaiting=off  DrvName=Advantech/PCI-1711  DrvAddress=4294967295  DrvOptions=zeros(1,0)  Channels=1  BitMode=2  InitialValue=0  FinalValue=0
      settings: AttributesFormatString=Advantech\nPCI-1711 [auto]
  wires:
  Constant/1 -> Digital Output/1

== system UpDownPendulum/Cart Position_Pendulum Angle/While Iterator Subsystem/latch for high ==
  Action Port : ActionPort  ActionType=case
  Constant : Constant  Value=4  OutDataTypeStr=double
  Digital Output : sldrtlib/Digital Output  SampleTime=-1  MaxMissedTicks=10  ShowMissedTicks=off  YieldWhenWaiting=off  DrvName=Advantech/PCI-1711  DrvAddress=4294967295  DrvOptions=zeros(1,0)  Channels=1  BitMode=2  InitialValue=0  FinalValue=0
      settings: AttributesFormatString=Advantech\nPCI-1711 [auto]
  wires:
  Constant/1 -> Digital Output/1

== system UpDownPendulum/Lower zone stabilization and crane control/Crane control/PID Controller  with D part filter ==
  In_1 : Inport
  D : Gain  Gain=D  SaturateOnIntegerOverflow=on  OutDataTypeStr=Inherit: Same as input  ParamDataTypeStr=Inherit: Same as input
  Derivative : Derivative
  Integral : TransferFcn  Numerator=[I]  Denominator=[1 0]
  Pendulum Velocity  Filter : TransferFcn  Numerator=[1e4]  Denominator=[1 70.7 1e4]
  Proportional : Gain  Gain=P  SaturateOnIntegerOverflow=on  OutDataTypeStr=Inherit: Same as input  ParamDataTypeStr=Inherit: Same as input
  Sum : Sum  Inputs=+++  SaturateOnIntegerOverflow=on  InputSameDT=on  OutDataTypeStr=Inherit: Same as first input
  Out_1 : Outport  InitialOutput=0
  wires:
  Pendulum Velocity  Filter/1 -> Sum/3
  D/1 -> Derivative/1
  Sum/1 -> Out_1/1
  In_1/1 -> D/1, Proportional/1, Integral/1
  Derivative/1 -> Pendulum Velocity  Filter/1
  Integral/1 -> Sum/2
  Proportional/1 -> Sum/1

== system UpDownPendulum/Lower zone stabilization and crane control/Crane control/PID1 Controller  with D part filter ==
  In_1 : Inport
  D : Gain  Gain=D  SaturateOnIntegerOverflow=on  OutDataTypeStr=Inherit: Same as input  ParamDataTypeStr=Inherit: Same as input
  Derivative : Derivative
  Integral : TransferFcn  Numerator=[I]  Denominator=[1 0]
  Pendulum Velocity  Filter : TransferFcn  Numerator=[1e4]  Denominator=[1 70.7 1e4]
  Proportional : Gain  Gain=P  SaturateOnIntegerOverflow=on  OutDataTypeStr=Inherit: Same as input  ParamDataTypeStr=Inherit: Same as input
  Sum : Sum  Inputs=+++  SaturateOnIntegerOverflow=on  InputSameDT=on  OutDataTypeStr=Inherit: Same as first input
  Out_1 : Outport  InitialOutput=0
  wires:
  Proportional/1 -> Sum/1
  Integral/1 -> Sum/2
  Derivative/1 -> Pendulum Velocity  Filter/1
  In_1/1 -> Integral/1, Proportional/1, D/1
  Sum/1 -> Out_1/1
  D/1 -> Derivative/1
  Pendulum Velocity  Filter/1 -> Sum/3

== system UpDownPendulum/Swing up and stabilization control/Inverted pendulum stabilization/PID Controller  with D part filter ==
  In_1 : Inport
  D : Gain  Gain=D  SaturateOnIntegerOverflow=on  OutDataTypeStr=Inherit: Same as input  ParamDataTypeStr=Inherit: Same as input
  Derivative : Derivative
  Integral : TransferFcn  Numerator=[I]  Denominator=[1 0]
  Pendulum Velocity  Filter : TransferFcn  Numerator=[1e4]  Denominator=[1 70.7 1e4]
  Proportional : Gain  Gain=P  SaturateOnIntegerOverflow=on  OutDataTypeStr=Inherit: Same as input  ParamDataTypeStr=Inherit: Same as input
  Sum : Sum  Inputs=+++  SaturateOnIntegerOverflow=on  InputSameDT=on  OutDataTypeStr=Inherit: Same as first input
  Out_1 : Outport  InitialOutput=0
  wires:
  Proportional/1 -> Sum/1
  Integral/1 -> Sum/2
  Derivative/1 -> Pendulum Velocity  Filter/1
  In_1/1 -> Integral/1, Proportional/1, D/1
  Sum/1 -> Out_1/1
  D/1 -> Derivative/1
  Pendulum Velocity  Filter/1 -> Sum/3

== system UpDownPendulum/Swing up and stabilization control/Inverted pendulum stabilization/PID1 Controller  with D part filter ==
  In_1 : Inport
  D : Gain  Gain=D  SaturateOnIntegerOverflow=on  OutDataTypeStr=Inherit: Same as input  ParamDataTypeStr=Inherit: Same as input
  Derivative : Derivative
  Integral : TransferFcn  Numerator=[I]  Denominator=[1 0]
  Pendulum Velocity  Filter : TransferFcn  Numerator=[1e4]  Denominator=[1 70.7 1e4]
  Proportional : Gain  Gain=P  SaturateOnIntegerOverflow=on  OutDataTypeStr=Inherit: Same as input  ParamDataTypeStr=Inherit: Same as input
  Sum : Sum  Inputs=+++  SaturateOnIntegerOverflow=on  InputSameDT=on  OutDataTypeStr=Inherit: Same as first input
  Out_1 : Outport  InitialOutput=0
  wires:
  Pendulum Velocity  Filter/1 -> Sum/3
  D/1 -> Derivative/1
  Sum/1 -> Out_1/1
  In_1/1 -> D/1, Proportional/1, Integral/1
  Derivative/1 -> Pendulum Velocity  Filter/1
  Integral/1 -> Sum/2
  Proportional/1 -> Sum/1

== system UpDownPendulum/Swing up and stabilization control/Swing up control + position control/EmptySubsystem ==

== system UpDownPendulum/Swing up and stabilization control/Swing up control + position control/Extra PI control for cart position ==
  position set point : Inport
  cart position : Inport  Port=2
  Add1 : Sum  Inputs=+-
  PID Controller  with D part filter : Subsystem  AncestorBlock=simulink_extras/Additional Linear/PID Controller  mask(PID Controller){P=0.5, I=0.2, D=0}
      mask prompts: P "Proportional:"; I "Integral:"; D "Derivative:"
      mask help:
      | Enter expressions for proportional, integral, and derivative terms.
      | P+I/s+Ds
      mask Help: This block implements a PID controller where parameters are entered for the Proportional, Integral and Derivative terms. Unmask this block to see how it works. The derivative term is implemented using a true derivative block.
      mask Display: disp('PID')
  extra control signal : Outport
  wires:
  Add1/1 -> PID Controller  with D part filter/1(In_1)
  position set point/1 -> Add1/1
  PID Controller  with D part filter/1(Out_1) -> extra control signal/1
  cart position/1 -> Add1/2

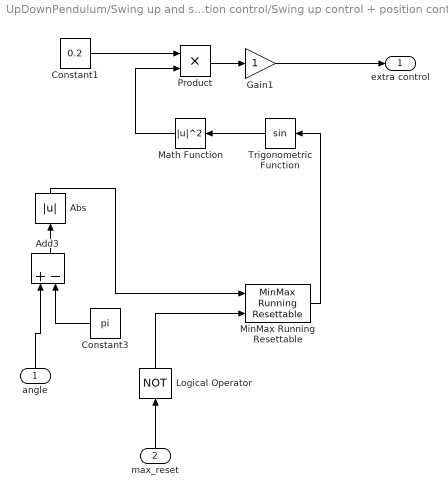
== system UpDownPendulum/Swing up and stabilization control/Swing up control + position control/Extra voltage depending on pendulum position,  slow start and slow finish ==
  angle : Inport
  max_reset : Inport  Port=2
  Abs : Abs
  Add3 : Sum  Inputs=+-
  Constant1 : Constant  Value=0.2
  Constant3 : Constant  Value=pi
  Gain1 : Gain
  Logical Operator : Logic  Operator=NOT  AllPortsSameDT=off  OutDataTypeStr=boolean
  Math Function : Math  Operator=magnitude^2  SaturateOnIntegerOverflow=on
  MinMax Running Resettable : simulink/Math Operations/MinMax Running Resettable  Function=max  vinit=0.0
  Product : Product  RndMeth=Zero
  Trigonometric Function : Trigonometry
  extra control : Outport
  wires:
  Product/1 -> Gain1/1
  Constant1/1 -> Product/1
  Constant3/1 -> Add3/2
  Add3/1 -> Abs/1
  Abs/1 -> MinMax Running Resettable/1
  Trigonometric Function/1 -> Math Function/1
  Gain1/1 -> extra control/1
  Math Function/1 -> Product/2
  angle/1 -> Add3/1
  max_reset/1 -> Logical Operator/1
  MinMax Running Resettable/1 -> Trigonometric Function/1
  Logical Operator/1 -> MinMax Running Resettable/2

== system UpDownPendulum/Swing up and stabilization control/Swing up control + position control/Upper / lower zone detection ==
  angle : Inport
  Compare To Constant : simulink/Logic and Bit Operations/Compare To Constant  relop=<=  const=pi/2  OutDataTypeStr=uint8  ZeroCross=off
  Compare To Constant1 : simulink/Logic and Bit Operations/Compare To Constant  relop=>=  const=pi/2+pi  OutDataTypeStr=uint8  ZeroCross=off
  Logical Operator : Logic  Operator=OR  AllPortsSameDT=off  OutDataTypeStr=boolean
  upper zone detection : Outport
  wires:
  Compare To Constant/1 -> Logical Operator/1
  Compare To Constant1/1 -> Logical Operator/2
  angle/1 -> Compare To Constant/1, Compare To Constant1/1
  Logical Operator/1 -> upper zone detection/1

== system UpDownPendulum/Swing up and stabilization control/Swing up control + position control/Voltage sign switching depending on pendulum position ==
  angular velocity : Inport
  control voltage : Inport  Port=2
  upper / lower zone detection : Inport  Port=3
  Enable : EnablePort
  Gain : Gain  Gain=-1
  Gain2 : Gain  Gain=-1
  upper or lower : Switch  Criteria=u2 > Threshold  Threshold=0.5
  zero velocity : Switch
  control voltage to the motor : Outport
  wires:
  Gain/1 -> upper or lower/3
  zero velocity/1 -> upper or lower/1, Gain/1
  control voltage/1 -> zero velocity/1, Gain2/1
  Gain2/1 -> zero velocity/3
  angular velocity/1 -> zero velocity/2
  upper or lower/1 -> control voltage to the motor/1
  upper / lower zone detection/1 -> upper or lower/2

== system UpDownPendulum/Swing up and stabilization control/Swing up control + position control/first move ==
  pulse : Inport
  Add1 : Sum  Inputs=+-
  Product : Product  RndMeth=Zero
  control v2 : Constant  Value=0.4
  initialization : Outport
  wires:
  control v2/1 -> Add1/1, Product/1
  Product/1 -> Add1/2
  pulse/1 -> Product/2
  Add1/1 -> initialization/1

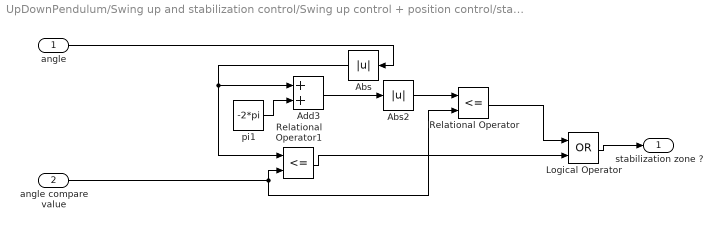
== system UpDownPendulum/Swing up and stabilization control/Swing up control + position control/stabilization zone detection  ==
  angle : Inport
  angle compare value : Inport  Port=2
  Abs : Abs
  Abs2 : Abs
  Add3 : Sum
  Logical Operator : Logic  Operator=OR  AllPortsSameDT=off  OutDataTypeStr=boolean
  Relational Operator : RelationalOperator  Operator=<=  OutDataTypeStr=boolean
  Relational Operator1 : RelationalOperator  Operator=<=  OutDataTypeStr=boolean
  pi1 : Constant  Value=-2*pi
  stabilization zone ? : Outport
  wires:
  Abs/1 -> Add3/1, Relational Operator1/1
  Relational Operator1/1 -> Logical Operator/2
  pi1/1 -> Add3/2
  Add3/1 -> Abs2/1
  Relational Operator/1 -> Logical Operator/1
  Abs2/1 -> Relational Operator/1
  angle/1 -> Abs/1
  Logical Operator/1 -> stabilization zone ?/1
  angle compare value/1 -> Relational Operator1/2, Relational Operator/2

== system UpDownPendulum/Cart Position_Pendulum Angle/While Iterator Subsystem/Reset/Subsystem ==
  In1 : Inport
  Constant1 : Constant  Value=7  OutDataTypeStr=double
  Digital Output : sldrtlib/Digital Output  SampleTime=-1  MaxMissedTicks=10  ShowMissedTicks=off  YieldWhenWaiting=off  DrvName=Advantech/PCI-1711  DrvAddress=4294967295  DrvOptions=zeros(1,0)  Channels=[1 2 3]  BitMode=2  InitialValue=0  FinalValue=0
      settings: AttributesFormatString=Advantech\nPCI-1711 [auto]
  Out1 : Outport
  wires:
  In1/1 -> Digital Output/1
  Constant1/1 -> Out1/1

== system UpDownPendulum/Swing up and stabilization control/Swing up control + position control/Extra PI control for cart position/PID Controller  with D part filter ==
  In_1 : Inport
  D : Gain  Gain=D  SaturateOnIntegerOverflow=on  OutDataTypeStr=Inherit: Same as input  ParamDataTypeStr=Inherit: Same as input
  Derivative : Derivative
  Integral : TransferFcn  Numerator=[I]  Denominator=[1 0]
  Pendulum Velocity  Filter : TransferFcn  Numerator=[1e4]  Denominator=[1 70.7 1e4]
  Proportional : Gain  Gain=P  SaturateOnIntegerOverflow=on  OutDataTypeStr=Inherit: Same as input  ParamDataTypeStr=Inherit: Same as input
  Sum : Sum  Inputs=+++  SaturateOnIntegerOverflow=on  InputSameDT=on  OutDataTypeStr=Inherit: Same as first input
  Out_1 : Outport  InitialOutput=0
  wires:
  Proportional/1 -> Sum/1
  Integral/1 -> Sum/2
  Derivative/1 -> Pendulum Velocity  Filter/1
  In_1/1 -> Integral/1, Proportional/1, D/1
  Sum/1 -> Out_1/1
  D/1 -> Derivative/1
  Pendulum Velocity  Filter/1 -> Sum/3
